simulink model "pscIJ"  (R2015a)
settings: Solver=ode45  SolverMode=SingleTasking  StartTime=0.0  StopTime=5  RelTol=1e-3
values from neighbouring files (symbols this model uses):
  B = [1;0]    [Lyglobal.m]
  Y = [Y yk]    [PDCtracking.m]
undefined symbols (not defined in the file or in its folder): J, kd, kp, smiData, X, Z
libraries: sm_lib x35, nesl_utility x13
(part 2 of 2)

== system pscIJ/Modelo 3-D con control pd/x1_Tercer_Arcticulacion_Rev1_1_RIGID ==
  ReferenceFrame : sm_lib/Frames and Transforms/Reference Frame
  Solid : sm_lib/Body Elements/Solid  InertiaType=Custom  Mass=smiData.Solid(5).mass  MassUnits=kg  CenterOfMass=smiData.Solid(5).CoM  CenterOfMassUnits=mm  MomentsOfInertia=smiData.Solid(5).MoI  MomentsOfInertiaUnits=kg*mm^2  ProductsOfInertia=smiData.Solid(5).PoI  ProductsOfInertiaUnits=kg*mm^2  DensityBased=on  Density=1000  DensityUnits=kg/m^3  DoExposeReferenceFrame=on  SerializedFrames=<Frames/>  GraphicType=FromGeometry  MarkerShape=Sphere  MarkerSize=10  GraphicVisPropType=SimpleVisualProperties  GraphicDiffuseColor=smiData.Solid(5).color  GraphicSpecularColor=[0.5 0.5 0.5 1.0]  GraphicAmbientColor=[0.15 0.15 0.15 1.0]  GraphicEmissiveColor=[0.0 0.0 0.0 1.0]  GraphicShininess=75  GraphicOpacity=smiData.Solid(5).opacity  GeometryShape=FromFile  RectangleSize=[1 1]  RectangleSizeUnits=m  BrickDimensions=[1 1 1]  BrickDimensionUnits=m  CylinderRadius=1  CylinderRadiusUnits=m  CylinderLength=1  CylinderLengthUnits=m  SphereRadius=1  SphereRadiusUnits=m  EllipsoidRadii=[1 1 1]  EllipsoidRadiiUnits=m  ExtrusionCrossSection=[1 1; -1 1; -1 -1; 1 -1]  ExtrusionCrossSectionUnits=m  ExtrusionLength=1  ExtrusionLengthUnits=m  PolygonNumSides=3  PolygonOuterRadius=1  PolygonOuterRadiusUnits=m  ExtGeomFileType=STEP  ExtGeomFileName=1 Tercer Arcticulacion Rev1_Predeterminado_sldprt.STEP  ExtGeomFileUnits=m  RevolutionCrossSection=[1 1; 1 -1; 2 -1; 2 1]  RevolutionCrossSectionUnits=m  RevolutionExtent=Full  RevolutionAngle=180  RevolutionAngleUnits=deg
  Transform : sm_lib/Frames and Transforms/Rigid Transform  TranslationMethod=Cartesian  TranslationStandardOffset=0  TranslationLengthUnit=m  TranslationStandardAxis=+Z  TranslationCartesianOffset=smiData.RigidTransform(1).translation  TranslationROffset=0  TranslationROffsetUnits=m  TranslationZOffset=0  TranslationZOffsetUnits=m  TranslationThetaOffset=0  TranslationThetaOffsetUnits=deg  RotationMethod=ArbitraryAxis  RotationAngleUnits=rad  RotationStandardAxis=+Z  RotationAngle=smiData.RigidTransform(1).angle  RotationArbitraryAxis=smiData.RigidTransform(1).axis  FollAlignAxisA=+X  BaseAlignAxisA=+Y  FollAlignAxisB=+Y  BaseAlignAxisB=+Z  RotationSequenceAxes=FollowerAxes  RotationSequence=XYX  RotationSequenceAngles=[0 0 0]  RotationSequenceAnglesUnits=deg  RotationMatrix=[1 0 0; 0 1 0; 0 0 1]
  Transform1 : sm_lib/Frames and Transforms/Rigid Transform  TranslationMethod=Cartesian  TranslationStandardOffset=0  TranslationLengthUnit=m  TranslationStandardAxis=+Z  TranslationCartesianOffset=smiData.RigidTransform(4).translation  TranslationROffset=0  TranslationROffsetUnits=m  TranslationZOffset=0  TranslationZOffsetUnits=m  TranslationThetaOffset=0  TranslationThetaOffsetUnits=deg  RotationMethod=ArbitraryAxis  RotationAngleUnits=rad  RotationStandardAxis=+Z  RotationAngle=smiData.RigidTransform(4).angle  RotationArbitraryAxis=smiData.RigidTransform(4).axis  FollAlignAxisA=+X  BaseAlignAxisA=+Y  FollAlignAxisB=+Y  BaseAlignAxisB=+Z  RotationSequenceAxes=FollowerAxes  RotationSequence=XYX  RotationSequenceAngles=[0 0 0]  RotationSequenceAnglesUnits=deg  RotationMatrix=[1 0 0; 0 1 0; 0 0 1]
  F1 : PMIOPort  Port=1  Side=Left
  F : PMIOPort  Port=2  Side=Right
  connections:
  Solid/RConn1 -- ReferenceFrame/RConn1 -- Transform/LConn1 -- Transform1/LConn1
  Transform/RConn1 -- F/RConn1
  Transform1/RConn1 -- F1/RConn1

== matlab function pscIJ/Cinematica Directa ==
  data: x output; q1 input; y output; z output; q2 input; q3 input; q4 input; q5 input; q6 input
function [x,y,z]= fcn(q1,q2,q3,q4,q5,q6)
 %segunda CD es de alex                                                                                          
% longitud en metros 
l1=0.1794;
l2=.08490;
l3=0.12580;
l4=0.16579+.083;
l5=0.03;
%%Pos= [l4*cos(q2)*cos(q3)*sin(q1) - l3*cos(q2)*sin(q1) - l2*sin(q1) + l5*cos(q1)*sin(q4)*sin(q5) - l4*sin(q1)*sin(q2)*sin(q3) + l5*cos(q2)*cos(q3)*cos(q5)*sin(q1) - l5*cos(q5)*sin(q1)*sin(q2)*sin(q3) - l5*cos(q2)*cos(q4)*sin(q1)*sin(q3)*sin(q5) - l5*cos(q3)*cos(q4)*sin(q1)*sin(q2)*sin(q5); l2*cos(q1) + l3*cos(q1)*cos(q2) - l4*cos(q1)*cos(q2)*cos(q3) + l4*cos(q1)*sin(q2)*sin(q3) + l5*sin(q1)*sin(q4)*sin(q5) - l5*cos(q1)*cos(q2)*cos(q3)*cos(q5) + l5*cos(q1)*cos(q5)*sin(q2)*sin(q3) + l5*cos(q1)*cos(q2)*cos(q4)*sin(q3)*sin(q5) + l5*cos(q1)*cos(q3)*cos(q4)*sin(q2)*sin(q5); l1 + l3*sin(q2) - l4*cos(q2)*sin(q3) - l4*cos(q3)*sin(q2) - l5*cos(q2)*cos(q5)*sin(q3) - l5*cos(q3)*cos(q5)*sin(q2) - l5*cos(q2)*cos(q3)*cos(q4)*sin(q5) + l5*cos(q4)*sin(q2)*sin(q3)*sin(q5)];
%%Pos=[-sin(q1)*(l2 - l4*cos(q2 + q3) + l3*cos(q2)); cos(q1)*(l2 - l4*cos(q2 + q3) + l3*cos(q2)); l1 - l4*sin(q2 + q3) + l3*sin(q2)]
%Pos=[cos(q1)*(l2 - l4*cos(q2 + q3) + l3*cos(q2)); 
%    sin(q1)*(l2 - l4*cos(q2 + q3) + l3*cos(q2)); 
%    l1 + l4*sin(q2 + q3) - l3*sin(q2)]
%%%Pos=[cos(q1)*(l2 + l4*cos(q2 + q3) + l3*cos(q2));
%%%    sin(q1)*(l2 + l4*cos(q2 + q3) + l3*cos(q2)); 
%%%    l1 + l4*sin(q2 + q3) + l3*sin(q2)]
Pos=[l2*cos(q1) + l3*cos(q1)*cos(q2) + l4*cos(q1)*cos(q2)*cos(q3) - l4*cos(q1)*sin(q2)*sin(q3) + l5*sin(q1)*sin(q4)*sin(q5) + l5*cos(q1)*cos(q2)*cos(q3)*cos(q5) - l5*cos(q1)*cos(q5)*sin(q2)*sin(q3) - l5*cos(q1)*cos(q2)*cos(q4)*sin(q3)*sin(q5) - l5*cos(q1)*cos(q3)*cos(q4)*sin(q2)*sin(q5);
    l2*sin(q1) + l3*cos(q2)*sin(q1) + l4*cos(q2)*cos(q3)*sin(q1) - l5*cos(q1)*sin(q4)*sin(q5) - l4*sin(q1)*sin(q2)*sin(q3) + l5*cos(q2)*cos(q3)*cos(q5)*sin(q1) - l5*cos(q5)*sin(q1)*sin(q2)*sin(q3) - l5*cos(q2)*cos(q4)*sin(q1)*sin(q3)*sin(q5) - l5*cos(q3)*cos(q4)*sin(q1)*sin(q2)*sin(q5); 
    l1 + l3*sin(q2) + l4*cos(q2)*sin(q3) + l4*cos(q3)*sin(q2) + l5*cos(q2)*cos(q5)*sin(q3) + l5*cos(q3)*cos(q5)*sin(q2) + l5*cos(q2)*cos(q3)*cos(q4)*sin(q5) - l5*cos(q4)*sin(q2)*sin(q3)*sin(q5)]

%cinemática directa 
%x = Pos(1);
%y = Pos(2); %signo (- )para que cambie el cuadrante 
%z = Pos(3);

x=Pos(1);
y=Pos(2);
z=Pos(3);

== matlab function pscIJ/Trayectorias Rev2 ==
  data: x output; t input; y output; z output
function [x,y,z]= fcn(t)
% % # circulo
  %wt= t*pi/7;
% % 
  %z = 0.1+.025*cos(wt);
  %x = 0.1+.025*sin(wt);
  %y = 0.30;

% %# Rosa polar 
% x_c=0.05; %% x_c y y_c representa el centro 
% y_c=0.1;
% r=0.02+0.05*sin(t);%% este es el radio de la figura
% x=x_c+r*sin(t);
% y=y_c+r*cos(t);
% z = 0.10;

% %# Rosa polar 3 petalos
x_c=0.05;
y_c=0.05;
r=0.02*sin(3*t); % 3 petalos
x=x_c+r*sin(t);
y=y_c+r*cos(t);
z = 0.4;%.40

% % %%%
% if(t<5)
%  y =0.15;
%  x = 0.1;
%  z = 0.1;
% elseif(t<10)
%  y =-0.15;
%  x = 0.1;
%  z = 0.05;
% elseif(t<15)
%  y =-0.15;
%  x = 0.06;
%  z = 0.1;
% elseif(t<20)
%  y =0.15;
%  x = 0.06;
%  z = 0.05;
% else(t<25)
%  y =0.15;
%  x = 0.1;
%  z = 0.1;
% end


%

== matlab function pscIJ/J06/Jaco ==
  data: q1 input; J output; q2 input; q3 input; q4 input; q5 input; q6 input
function J = fcn(q1,q2,q3,q4,q5,q6)
 %segunda CD es de alex                                                                                          
% longitud en metros 
l1=0.1794;
l2=.08490;
l3=0.12580;
l4=0.16579+.083;
l5=0.01786;

Z0=[0;0;1];
Z1=[-sin(q1);cos(q1);0];
Z2=[-sin(q1);cos(q1);0];
Z3=[-sin(q1);cos(q1);0];
Z4=[cos(q1)*cos(q2)*sin(q3)*sin(q4) - cos(q4)*sin(q1) + cos(q1)*cos(q3)*sin(q2)*sin(q4);
    cos(q1)*cos(q4) + cos(q2)*sin(q1)*sin(q3)*sin(q4) + cos(q3)*sin(q1)*sin(q2)*sin(q4);
    cos(q2 + q3)*sin(q4)];
Z5=[cos(q2 + q3)*cos(q1)*cos(q5) - sin(q5)*(sin(q1)*sin(q4) + cos(q1)*cos(q2)*cos(q4)*sin(q3) + cos(q1)*cos(q3)*cos(q4)*sin(q2))
    ;cos(q2 + q3)*cos(q5)*sin(q1) - sin(q5)*(cos(q2)*cos(q4)*sin(q1)*sin(q3) - cos(q1)*sin(q4) + cos(q3)*cos(q4)*sin(q1)*sin(q2))
    ;- sin(q2 + q3)*cos(q5) - cos(q2 + q3)*cos(q4)*sin(q5)];
Z6=[cos(q2 + q3)*cos(q1)*cos(q5) - sin(q5)*(sin(q1)*sin(q4) + cos(q1)*cos(q2)*cos(q4)*sin(q3) + cos(q1)*cos(q3)*cos(q4)*sin(q2))
    ; cos(q2 + q3)*cos(q5)*sin(q1) - sin(q5)*(cos(q2)*cos(q4)*sin(q1)*sin(q3) - cos(q1)*sin(q4) + cos(q3)*cos(q4)*sin(q1)*sin(q2))
    ;- sin(q2 + q3)*cos(q5) - cos(q2 + q3)*cos(q4)*sin(q5)];



A1=[l4*sin(q1)*sin(q2)*sin(q3) - l3*cos(q2)*sin(q1) - l4*cos(q2)*cos(q3)*sin(q1) - l5*cos(q1)*sin(q4)*sin(q5) - l2*sin(q1) - l5*cos(q2)*cos(q3)*cos(q5)*sin(q1) + l5*cos(q5)*sin(q1)*sin(q2)*sin(q3) + l5*cos(q2)*cos(q4)*sin(q1)*sin(q3)*sin(q5) + l5*cos(q3)*cos(q4)*sin(q1)*sin(q2)*sin(q5);
    l2*cos(q1) + l3*cos(q1)*cos(q2) + l4*cos(q1)*cos(q2)*cos(q3) - l4*cos(q1)*sin(q2)*sin(q3) - l5*sin(q1)*sin(q4)*sin(q5) + l5*cos(q1)*cos(q2)*cos(q3)*cos(q5) - l5*cos(q1)*cos(q5)*sin(q2)*sin(q3) - l5*cos(q1)*cos(q2)*cos(q4)*sin(q3)*sin(q5) - l5*cos(q1)*cos(q3)*cos(q4)*sin(q2)*sin(q5);
                                                                          0]
A2= [-cos(q1)*(l3*sin(q2) + l4*cos(q2)*sin(q3) + l4*cos(q3)*sin(q2) + l5*cos(q2)*cos(q5)*sin(q3) + l5*cos(q3)*cos(q5)*sin(q2) + l5*cos(q2)*cos(q3)*cos(q4)*sin(q5) - l5*cos(q4)*sin(q2)*sin(q3)*sin(q5));
    -sin(q1)*(l3*sin(q2) + l4*cos(q2)*sin(q3) + l4*cos(q3)*sin(q2) + l5*cos(q2)*cos(q5)*sin(q3) + l5*cos(q3)*cos(q5)*sin(q2) + l5*cos(q2)*cos(q3)*cos(q4)*sin(q5) - l5*cos(q4)*sin(q2)*sin(q3)*sin(q5));
     l4*sin(q2)*sin(q3) - l4*cos(q2)*cos(q3) - l3*cos(q2) - l5*cos(q2)*cos(q3)*cos(q5) + l5*cos(q5)*sin(q2)*sin(q3) + l5*cos(q2)*cos(q4)*sin(q3)*sin(q5) + l5*cos(q3)*cos(q4)*sin(q2)*sin(q5)]
 
A3= [ -cos(q1)*(l4*cos(q2)*sin(q3) + l4*cos(q3)*sin(q2) + l5*cos(q2)*cos(q5)*sin(q3) + l5*cos(q3)*cos(q5)*sin(q2) + l5*cos(q2)*cos(q3)*cos(q4)*sin(q5) - l5*cos(q4)*sin(q2)*sin(q3)*sin(q5));
     -sin(q1)*(l4*cos(q2)*sin(q3) + l4*cos(q3)*sin(q2) + l5*cos(q2)*cos(q5)*sin(q3) + l5*cos(q3)*cos(q5)*sin(q2) + l5*cos(q2)*cos(q3)*cos(q4)*sin(q5) - l5*cos(q4)*sin(q2)*sin(q3)*sin(q5));
      l4*sin(q2)*sin(q3) - l4*cos(q2)*cos(q3) - l5*cos(q2)*cos(q3)*cos(q5) + l5*cos(q5)*sin(q2)*sin(q3) + l5*cos(q2)*cos(q4)*sin(q3)*sin(q5) + l5*cos(q3)*cos(q4)*sin(q2)*sin(q5)]
 
     
A4=[-cos(q1)*(l4*cos(q2)*sin(q3) + l4*cos(q3)*sin(q2) + l5*cos(q2)*cos(q5)*sin(q3) + l5*cos(q3)*cos(q5)*sin(q2) + l5*cos(q2)*cos(q3)*cos(q4)*sin(q5) - l5*cos(q4)*sin(q2)*sin(q3)*sin(q5));
    -sin(q1)*(l4*cos(q2)*sin(q3) + l4*cos(q3)*sin(q2) + l5*cos(q2)*cos(q5)*sin(q3) + l5*cos(q3)*cos(q5)*sin(q2) + l5*cos(q2)*cos(q3)*cos(q4)*sin(q5) - l5*cos(q4)*sin(q2)*sin(q3)*sin(q5));
sin(q1)*(sin(q1)*(l2 + l3*cos(q2)) - l2*sin(q1) - l3*cos(q2)*sin(q1) - l4*cos(q2)*cos(q3)*sin(q1) - l5*cos(q1)*sin(q4)*sin(q5) + l4*sin(q1)*sin(q2)*sin(q3) - l5*cos(q2)*cos(q3)*cos(q5)*sin(q1) + l5*cos(q5)*sin(q1)*sin(q2)*sin(q3) + l5*cos(q2)*cos(q4)*sin(q1)*sin(q3)*sin(q5) + l5*cos(q3)*cos(q4)*sin(q1)*sin(q2)*sin(q5)) + cos(q1)*(cos(q1)*(l2 + l3*cos(q2)) - l2*cos(q1) - l3*cos(q1)*cos(q2) - l4*cos(q1)*cos(q2)*cos(q3) + l4*cos(q1)*sin(q2)*sin(q3) + l5*sin(q1)*sin(q4)*sin(q5) - l5*cos(q1)*cos(q2)*cos(q3)*cos(q5) + l5*cos(q1)*cos(q5)*sin(q2)*sin(q3) + l5*cos(q1)*cos(q2)*cos(q4)*sin(q3)*sin(q5) + l5*cos(q1)*cos(q3)*cos(q4)*sin(q2)*sin(q5))]

A5=[-cos(q1)*(l4*cos(q2)*sin(q3) - l4*sin(q2 + q3) + l4*cos(q3)*sin(q2) + l5*cos(q2)*cos(q5)*sin(q3) + l5*cos(q3)*cos(q5)*sin(q2) + l5*cos(q2)*cos(q3)*cos(q4)*sin(q5) - l5*cos(q4)*sin(q2)*sin(q3)*sin(q5));
    -sin(q1)*(l4*cos(q2)*sin(q3) - l4*sin(q2 + q3) + l4*cos(q3)*sin(q2) + l5*cos(q2)*cos(q5)*sin(q3) + l5*cos(q3)*cos(q5)*sin(q2) + l5*cos(q2)*cos(q3)*cos(q4)*sin(q5) - l5*cos(q4)*sin(q2)*sin(q3)*sin(q5));
    cos(q1)*(cos(q1)*(l2 + l4*cos(q2 + q3) + l3*cos(q2)) - l2*cos(q1) - l3*cos(q1)*cos(q2) - l4*cos(q1)*cos(q2)*cos(q3) + l4*cos(q1)*sin(q2)*sin(q3) + l5*sin(q1)*sin(q4)*sin(q5) - l5*cos(q1)*cos(q2)*cos(q3)*cos(q5) + l5*cos(q1)*cos(q5)*sin(q2)*sin(q3) + l5*cos(q1)*cos(q2)*cos(q4)*sin(q3)*sin(q5) + l5*cos(q1)*cos(q3)*cos(q4)*sin(q2)*sin(q5)) + sin(q1)*(sin(q1)*(l2 + l4*cos(q2 + q3) + l3*cos(q2)) - l2*sin(q1) - l3*cos(q2)*sin(q1) - l4*cos(q2)*cos(q3)*sin(q1) - l5*cos(q1)*sin(q4)*sin(q5) + l4*sin(q1)*sin(q2)*sin(q3) - l5*cos(q2)*cos(q3)*cos(q5)*sin(q1) + l5*cos(q5)*sin(q1)*sin(q2)*sin(q3) + l5*cos(q2)*cos(q4)*sin(q1)*sin(q3)*sin(q5) + l5*cos(q3)*cos(q4)*sin(q1)*sin(q2)*sin(q5))]
A6=[-cos(q1)*(l4*cos(q2)*sin(q3) - l4*sin(q2 + q3) + l4*cos(q3)*sin(q2) + l5*cos(q2)*cos(q5)*sin(q3) + l5*cos(q3)*cos(q5)*sin(q2) + l5*cos(q2)*cos(q3)*cos(q4)*sin(q5) - l5*cos(q4)*sin(q2)*sin(q3)*sin(q5));
    -sin(q1)*(l4*cos(q2)*sin(q3) - l4*sin(q2 + q3) + l4*cos(q3)*sin(q2) + l5*cos(q2)*cos(q5)*sin(q3) + l5*cos(q3)*cos(q5)*sin(q2) + l5*cos(q2)*cos(q3)*cos(q4)*sin(q5) - l5*cos(q4)*sin(q2)*sin(q3)*sin(q5));
    cos(q1)*(cos(q1)*(l2 + l4*cos(q2 + q3) + l3*cos(q2)) - l2*cos(q1) - l3*cos(q1)*cos(q2) - l4*cos(q1)*cos(q2)*cos(q3) + l4*cos(q1)*sin(q2)*sin(q3) + l5*sin(q1)*sin(q4)*sin(q5) - l5*cos(q1)*cos(q2)*cos(q3)*cos(q5) + l5*cos(q1)*cos(q5)*sin(q2)*sin(q3) + l5*cos(q1)*cos(q2)*cos(q4)*sin(q3)*sin(q5) + l5*cos(q1)*cos(q3)*cos(q4)*sin(q2)*sin(q5)) + sin(q1)*(sin(q1)*(l2 + l4*cos(q2 + q3) + l3*cos(q2)) - l2*sin(q1) - l3*cos(q2)*sin(q1) - l4*cos(q2)*cos(q3)*sin(q1) - l5*cos(q1)*sin(q4)*sin(q5) + l4*sin(q1)*sin(q2)*sin(q3) - l5*cos(q2)*cos(q3)*cos(q5)*sin(q1) + l5*cos(q5)*sin(q1)*sin(q2)*sin(q3) + l5*cos(q2)*cos(q4)*sin(q1)*sin(q3)*sin(q5) + l5*cos(q3)*cos(q4)*sin(q1)*sin(q2)*sin(q5))]


j11=[A1 A2 A3]
j12=[A4 A5 A6]
j21=[Z0 Z1 Z2]
j22=[Z3 Z4 Z5]
% j21=[ 0, -sin(q1), -sin(q1);0,  cos(q1),  cos(q1); 1,        0,        0];
% j12=[ -cos(q1)*(l4*cos(q2)*sin(q3) + l4*cos(q3)*sin(q2) + l5*cos(q2)*cos(q5)*sin(q3) + l5*cos(q3)*cos(q5)*sin(q2) + l5*cos(q2)*cos(q3)*cos(q4)*sin(q5) - l5*cos(q4)*sin(q2)*sin(q3)*sin(q5)), -l5*cos(q1)*(cos(q2)*cos(q5)*sin(q3) + cos(q3)*cos(q5)*sin(q2) + cos(q2)*cos(q3)*cos(q4)*sin(q5) - cos(q4)*sin(q2)*sin(q3)*sin(q5)), -l5*cos(q1)*(cos(q2)*cos(q5)*sin(q3) + cos(q3)*cos(q5)*sin(q2) + cos(q2)*cos(q3)*cos(q4)*sin(q5) - cos(q4)*sin(q2)*sin(q3)*sin(q5));
%     -sin(q1)*(l4*cos(q2)*sin(q3) + l4*cos(q3)*sin(q2) + l5*cos(q2)*cos(q5)*sin(q3) + l5*cos(q3)*cos(q5)*sin(q2) + l5*cos(q2)*cos(q3)*cos(q4)*sin(q5) - l5*cos(q4)*sin(q2)*sin(q3)*sin(q5)), -l5*sin(q1)*(cos(q2)*cos(q5)*sin(q3) + cos(q3)*cos(q5)*sin(q2) + cos(q2)*cos(q3)*cos(q4)*sin(q5) - cos(q4)*sin(q2)*sin(q3)*sin(q5)), -l5*sin(q1)*(cos(q2)*cos(q5)*sin(q3) + cos(q3)*cos(q5)*sin(q2) + cos(q2)*cos(q3)*cos(q4)*sin(q5) - cos(q4)*sin(q2)*sin(q3)*sin(q5));
%      l4*sin(q2)*sin(q3) - l4*cos(q2)*cos(q3) - l5*cos(q2)*cos(q3)*cos(q5) + l5*cos(q5)*sin(q2)*sin(q3) + l5*cos(q2)*cos(q4)*sin(q3)*sin(q5) + l5*cos(q3)*cos(q4)*sin(q2)*sin(q5),   l5*cos(q5)*sin(q2)*sin(q3) - l5*cos(q2)*cos(q3)*cos(q5) + l5*cos(q2)*cos(q4)*sin(q3)*sin(q5) + l5*cos(q3)*cos(q4)*sin(q2)*sin(q5),   l5*cos(q5)*sin(q2)*sin(q3) - l5*cos(q2)*cos(q3)*cos(q5) + l5*cos(q2)*cos(q4)*sin(q3)*sin(q5) + l5*cos(q3)*cos(q4)*sin(q2)*sin(q5)]
% 
%        
% 
% j22=[ -sin(q1), cos(q1)*cos(q2)*sin(q3)*sin(q4) - cos(q4)*sin(q1) + cos(q1)*cos(q3)*sin(q2)*sin(q4), cos(q2 + q3)*cos(q1)*cos(q5) - sin(q5)*(sin(q1)*sin(q4) + cos(q1)*cos(q2)*cos(q4)*sin(q3) + cos(q1)*cos(q3)*cos(q4)*sin(q2));
%      cos(q1), cos(q1)*cos(q4) + cos(q2)*sin(q1)*sin(q3)*sin(q4) + cos(q3)*sin(q1)*sin(q2)*sin(q4), cos(q2 + q3)*cos(q5)*sin(q1) - sin(q5)*(cos(q2)*cos(q4)*sin(q1)*sin(q3) - cos(q1)*sin(q4) + cos(q3)*cos(q4)*sin(q1)*sin(q2));
%              0,                                                                cos(q2 + q3)*sin(q4),                                                                        - sin(q2 + q3)*cos(q5) - cos(q2 + q3)*cos(q4)*sin(q5)]
 


J=[j11 j12;j21 j22];

== matlab function pscIJ/Cinematica Inversa  ==
  data: Q1 output; x input; Q2 output; Q3 output; y input; z input; Q4 output; Q5 output; Q6 output
function [Q1,Q2,Q3,Q4,Q5,Q6] = fcn(x,y,z)
l1=0.1794;
l2=0.08490;
l3=0.12580;
l4=0.16579+.083;
l5=0.03;


%%%codo Arriba
r=sqrt(x^2+y^2);
ca=r-l2; %%
co=z-l1; %%
Q1 = atan2(y,x);
hi=sqrt(ca^2+co^2);
C3 =((-hi^2+l3^2+l4^2)/(-2*l4*l3));
Q3= atan2(sqrt(1-C3^2),C3); %%Codo Arriba
Q2=atan2(co,ca)-atan2(l4*sin(Q3),l3+l4*cos(Q3));


Q4=atan2(cos(Q1),sin(Q2+Q3)*sin(Q1))
Q5=atan2(-sqrt(1-(cos(Q2+Q3)*cos(Q1))),cos(Q2+Q3)*cos(Q1))
Q6=atan2(sin(Q2+Q3),cos(Q2+Q3)*cos(Q1))

== matlab function pscIJ/Modelo 3-D con control pd/PD puntual ==
  data: qd input; y output; qpa input; qa input; e output
function [y,e] = fcn(qd,qpa,qa)
%Pd  sin tacking  
%qa=[0;0;0;0;0;0]

KP=[21.6;56;5.2;5;4;3]
KD=[4.82;10.22;1;.5;.4;.3]
e=[(qd(1)-qa(1));(qd(2)-qa(2));(qd(3)-qa(3));(qd(4)-qa(4));(qd(5)-qa(5));(qd(6)-qa(6))];
u=[(KP(1)*e(1)-KD(1)*qpa(1));(KP(2)*e(2)-KD(2)*qpa(2));(KP(3)*e(3)-KD(3)*qpa(3));(KP(4)*e(4)-KD(4)*qpa(4));(KP(5)*e(5)-KD(5)*qpa(5));(KP(6)*e(6)-KD(6)*qpa(5))]

y = u;
